simulink model "Aenea_model"  (R2020b)
settings: Solver=FixedStepDiscrete  StartTime=0.0  StopTime=10.0  FixedStep=0.02  RelTol=1e-3
undefined symbols (not defined in the file): attuatore_Amax, attuatore_Amin, attuatore_Emax, attuatore_Emin, attuatore_Rmax, attuatore_Rmin, attuatore_Tmax, attuatore_Tmin, bias, DiscIntNeverNeededParam, interventoA_05, interventoA_1, interventoE_05, interventoE_1, interventoT, inv_A, inv_comp_h, inv_E, inv_R, inv_T, K_AW_B_AP_quota, K_AW_B_becc, K_AW_B_imb, K_AW_B_roll, K_imb_inv, Kd_h_app, Kd_h_flare, Ki_AP_quota_select, Ki_AP_rotta, Ki_AP_vel, Ki_becch, Ki_h_app, Ki_h_cruise, Ki_h_flare, Ki_roll, Kp_AP_quota_hold_h, Kp_AP_quota_hold_l, Kp_AP_quota_select, Kp_AP_rotta, Kp_AP_vel, Kp_becch, Kp_comp_h, Kp_h_app_max, Kp_h_app_min, Kp_h_cruise, Kp_h_flare, Kp_imb, Kp_p, Kp_q, Kp_roll, Kp_Rotta_ATO, Newton, phi_max, phi_min, pwm_aileron_max, pwm_aileron_min, pwm_elevator_max, pwm_elevator_min, pwm_rudder_max, pwm_rudder_min ... (+19)
libraries: simulink_extras x41, slpidlib x8, simulink x6, dspsigops x4, arduinolib x3, svdutilitieslib x3, aerolibtransform2sys x2, aerolibtransform2 x2, aerosimlib x2, cstblocks x1
(part 5 of 7)

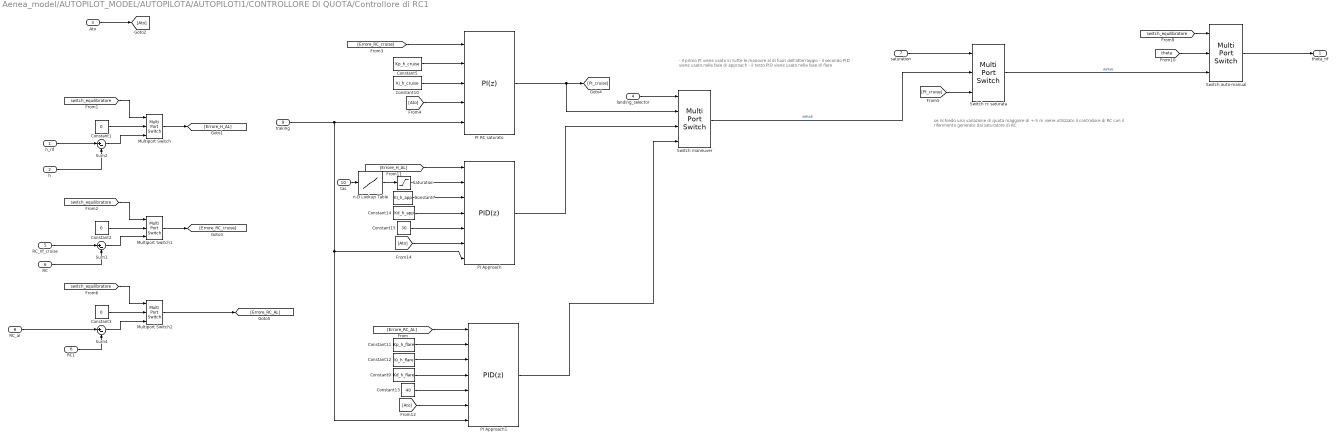
== system Aenea_model/AUTOPILOT_MODEL/AUTOPILOTA/AUTOPILOTI1/CONTROLLORE DI QUOTA/Controllore di RC1 ==
  note: - il primo PI viene usato in tutte le manovre al di fuori dell'atterraggio
      | - il secondo PID viene usato nella fase di approach
      | - il terzo PID viene usato nella fase di flare
  note: se richiedo una variazione di quota maggiore di +-5 m viene utilizzato il controllore di RC
      | con il riferimento generato dal saturatore di RC
  h_rif : Inport
  h : Inport  Port=2
  "Ato " : Inport  Port=3
  landing_selector : Inport  Port=4
  RC_rif_cruise : Inport  Port=5
  RC : Inport  Port=6
  saturation : Inport  Port=7
  "RC_al " : Inport  Port=8
  traking : Inport  Port=9
  tas : Inport  Port=10
  Constant1 : Constant  Value=0  SampleTime=t_AP
  Constant10 : Constant  Value=Ki_h_cruise  SampleTime=t_AP
  Constant11 : Constant  Value=Kp_h_flare  SampleTime=0.02
  Constant12 : Constant  Value=Ki_h_flare  SampleTime=0.02
  Constant13 : Constant  Value=40  SampleTime=0.02
  Constant14 : Constant  Value=Kd_h_app  SampleTime=0.02
  Constant15 : Constant  Value=30  SampleTime=0.02
  Constant2 : Constant  Value=0  SampleTime=t_AP
  Constant3 : Constant  Value=0  SampleTime=t_AP
  Constant5 : Constant  Value=Kp_h_cruise  SampleTime=t_AP
  Constant7 : Constant  Value=Ki_h_app  SampleTime=0.02
  Constant9 : Constant  Value=Kd_h_flare  SampleTime=0.02
  Multiport Switch : MultiPortSwitch  DataPortOrder=Zero-based contiguous  Inputs=2  zeroidx=on
  Multiport Switch1 : MultiPortSwitch  DataPortOrder=Zero-based contiguous  Inputs=2  zeroidx=on
  Multiport Switch2 : MultiPortSwitch  DataPortOrder=Zero-based contiguous  Inputs=2  zeroidx=on
  PI Approach : slpidlib/PID Controller  Controller=PID  Form=Parallel  TimeDomain=Discrete-time  UseExternalTs=off  SampleTime=0.02  IntegratorMethod=Forward Euler  FilterMethod=Forward Euler  ControllerParametersSource=external  P=1  I=1  D=0  UseFilter=on  N=100  TunerSelectOption=Transfer Function Based (PID Tuner App)  InitialConditionSource=internal  InitialConditionForIntegrator=0  InitialConditionForFilter=0  DifferentiatorICPrevScaledInput=0  ExternalReset=rising  TrackingMode=on  Kt=1  LimitOutput=off  SatLimitsSource=internal  UpperSaturationLimit=0.7  LowerSaturationLimit=-0.7  LinearizeAsGain=off  AntiWindupMode=back-calculation  Kb=1  POutMin=[]  POutMax=[]  IOutMin=[]  IOutMax=[]  DOutMin=[]  DOutMax=[]  NOutMin=[]  NOutMax=[]  SumOutMin=[]  SumOutMax=[]  SaturationOutMin=[]  SaturationOutMax=[]  PParamMin=[]  PParamMax=[]  IParamMin=[]  IParamMax=[]  DParamMin=[]  DParamMax=[]  NParamMin=[]  NParamMax=[]  KbParamMin=[]  KbParamMax=[]  KtParamMin=[]  KtParamMax=[]  KbOutMin=[]  KbOutMax=[]  KtOutMin=[]  KtOutMax=[]  IntegratorOutMin=[]  IntegratorOutMax=[]  FilterOutMin=[]  FilterOutMax=[]  SumI1OutMin=[]  SumI1OutMax=[]  SumI2OutMin=[]  SumI2OutMax=[]  SumI3OutMin=[]  SumI3OutMax=[]  SumI4OutMin=[]  SumI4OutMax=[]  SumDOutMin=[]  SumDOutMax=[]  DifferentiatorOutMin=[]  DifferentiatorOutMax=[]  FilterDiffOutCoefMin=[]  FilterDiffOutCoefMax=[]  ReciprocalOutMin=[]  ReciprocalOutMax=[]  SumDenOutMin=[]  SumDenOutMax=[]  SumNumOutMin=[]  SumNumOutMax=[]  DivideOutMin=[]  DivideOutMax=[]  UdiffTsProdOutMin=[]  UdiffTsProdOutMax=[]  NTsProdOutMin=[]  NTsProdOutMax=[]  UintegralTsProdOutMin=[]  UintegralTsProdOutMax=[]  UngainTsProdOutMin=[]  UngainTsProdOutMax=[]  IntegratorContinuousStateAttributes=''  IntegratorStateMustResolveToSignalObject=off  IntegratorRTWStateStorageClass=Auto  FilterContinuousStateAttributes=''  FilterStateMustResolveToSignalObject=off  FilterRTWStateStorageClass=Auto  ParallelPVariant=ExternalParameters  IdealPVariant=Disabled  IVariant=ExternalParameters  DVariant=ExternalParameters  IntegratorVariant=Discrete  SatVariant=Disabled  AWVariant=Passthrough  PCopyVariant=Disabled  TRVariant=Enabled  FdbkBlocksVariant=Forward  IdealPFdbkVariant=Disabled  SatFdbkVariant=Disabled  DerivativeFilterVariant=ForwardEulerFilter  NVariant=ExternalParameters  NCopyVariant=Disabled  FilterICVariant=InternalICsFilter  IntegratorICVariant=InternalICs  ExternalResetVariant=ExternalReset  TRSumVariant=TrackingMode  SumFdbkVariant=Disabled  SumVariant=Sum_PID  TsampFilterVariant=InternalTs  TsampNgainVariant=Passthrough  TsampIntegralVariant=Passthrough  ExternalSaturationOutDataTypeStr=Inherit: Same as second input
  PI Approach1 : slpidlib/PID Controller  Controller=PID  Form=Parallel  TimeDomain=Discrete-time  UseExternalTs=off  SampleTime=0.02  IntegratorMethod=Forward Euler  FilterMethod=Forward Euler  ControllerParametersSource=external  P=1  I=1  D=0  UseFilter=on  N=100  TunerSelectOption=Transfer Function Based (PID Tuner App)  InitialConditionSource=internal  InitialConditionForIntegrator=0  InitialConditionForFilter=0  DifferentiatorICPrevScaledInput=0  ExternalReset=rising  TrackingMode=on  Kt=1  LimitOutput=off  SatLimitsSource=internal  UpperSaturationLimit=0.7  LowerSaturationLimit=-0.7  LinearizeAsGain=off  AntiWindupMode=back-calculation  Kb=1  POutMin=[]  POutMax=[]  IOutMin=[]  IOutMax=[]  DOutMin=[]  DOutMax=[]  NOutMin=[]  NOutMax=[]  SumOutMin=[]  SumOutMax=[]  SaturationOutMin=[]  SaturationOutMax=[]  PParamMin=[]  PParamMax=[]  IParamMin=[]  IParamMax=[]  DParamMin=[]  DParamMax=[]  NParamMin=[]  NParamMax=[]  KbParamMin=[]  KbParamMax=[]  KtParamMin=[]  KtParamMax=[]  KbOutMin=[]  KbOutMax=[]  KtOutMin=[]  KtOutMax=[]  IntegratorOutMin=[]  IntegratorOutMax=[]  FilterOutMin=[]  FilterOutMax=[]  SumI1OutMin=[]  SumI1OutMax=[]  SumI2OutMin=[]  SumI2OutMax=[]  SumI3OutMin=[]  SumI3OutMax=[]  SumI4OutMin=[]  SumI4OutMax=[]  SumDOutMin=[]  SumDOutMax=[]  DifferentiatorOutMin=[]  DifferentiatorOutMax=[]  FilterDiffOutCoefMin=[]  FilterDiffOutCoefMax=[]  ReciprocalOutMin=[]  ReciprocalOutMax=[]  SumDenOutMin=[]  SumDenOutMax=[]  SumNumOutMin=[]  SumNumOutMax=[]  DivideOutMin=[]  DivideOutMax=[]  UdiffTsProdOutMin=[]  UdiffTsProdOutMax=[]  NTsProdOutMin=[]  NTsProdOutMax=[]  UintegralTsProdOutMin=[]  UintegralTsProdOutMax=[]  UngainTsProdOutMin=[]  UngainTsProdOutMax=[]  IntegratorContinuousStateAttributes=''  IntegratorStateMustResolveToSignalObject=off  IntegratorRTWStateStorageClass=Auto  FilterContinuousStateAttributes=''  FilterStateMustResolveToSignalObject=off  FilterRTWStateStorageClass=Auto  ParallelPVariant=ExternalParameters  IdealPVariant=Disabled  IVariant=ExternalParameters  DVariant=ExternalParameters  IntegratorVariant=Discrete  SatVariant=Disabled  AWVariant=Passthrough  PCopyVariant=Disabled  TRVariant=Enabled  FdbkBlocksVariant=Forward  IdealPFdbkVariant=Disabled  SatFdbkVariant=Disabled  DerivativeFilterVariant=ForwardEulerFilter  NVariant=ExternalParameters  NCopyVariant=Disabled  FilterICVariant=InternalICsFilter  IntegratorICVariant=InternalICs  ExternalResetVariant=ExternalReset  TRSumVariant=TrackingMode  SumFdbkVariant=Disabled  SumVariant=Sum_PID  TsampFilterVariant=InternalTs  TsampNgainVariant=Passthrough  TsampIntegralVariant=Passthrough  ExternalSaturationOutDataTypeStr=Inherit: Same as second input
  PI RC saturato : slpidlib/PID Controller  Controller=PI  Form=Parallel  TimeDomain=Discrete-time  UseExternalTs=off  SampleTime=0.02  IntegratorMethod=Forward Euler  FilterMethod=Forward Euler  ControllerParametersSource=external  P=1  I=1  D=0  UseFilter=on  N=100  TunerSelectOption=Transfer Function Based (PID Tuner App)  InitialConditionSource=internal  InitialConditionForIntegrator=0  InitialConditionForFilter=0  DifferentiatorICPrevScaledInput=0  ExternalReset=rising  TrackingMode=on  Kt=1  LimitOutput=off  SatLimitsSource=internal  UpperSaturationLimit=0.7  LowerSaturationLimit=-0.7  LinearizeAsGain=off  AntiWindupMode=back-calculation  Kb=1  POutMin=[]  POutMax=[]  IOutMin=[]  IOutMax=[]  DOutMin=[]  DOutMax=[]  NOutMin=[]  NOutMax=[]  SumOutMin=[]  SumOutMax=[]  SaturationOutMin=[]  SaturationOutMax=[]  PParamMin=[]  PParamMax=[]  IParamMin=[]  IParamMax=[]  DParamMin=[]  DParamMax=[]  NParamMin=[]  NParamMax=[]  KbParamMin=[]  KbParamMax=[]  KtParamMin=[]  KtParamMax=[]  KbOutMin=[]  KbOutMax=[]  KtOutMin=[]  KtOutMax=[]  IntegratorOutMin=[]  IntegratorOutMax=[]  FilterOutMin=[]  FilterOutMax=[]  SumI1OutMin=[]  SumI1OutMax=[]  SumI2OutMin=[]  SumI2OutMax=[]  SumI3OutMin=[]  SumI3OutMax=[]  SumI4OutMin=[]  SumI4OutMax=[]  SumDOutMin=[]  SumDOutMax=[]  DifferentiatorOutMin=[]  DifferentiatorOutMax=[]  FilterDiffOutCoefMin=[]  FilterDiffOutCoefMax=[]  ReciprocalOutMin=[]  ReciprocalOutMax=[]  SumDenOutMin=[]  SumDenOutMax=[]  SumNumOutMin=[]  SumNumOutMax=[]  DivideOutMin=[]  DivideOutMax=[]  UdiffTsProdOutMin=[]  UdiffTsProdOutMax=[]  NTsProdOutMin=[]  NTsProdOutMax=[]  UintegralTsProdOutMin=[]  UintegralTsProdOutMax=[]  UngainTsProdOutMin=[]  UngainTsProdOutMax=[]  IntegratorContinuousStateAttributes=''  IntegratorStateMustResolveToSignalObject=off  IntegratorRTWStateStorageClass=Auto  FilterContinuousStateAttributes=''  FilterStateMustResolveToSignalObject=off  FilterRTWStateStorageClass=Auto  ParallelPVariant=ExternalParameters  IdealPVariant=Disabled  IVariant=ExternalParameters  DVariant=Disabled  IntegratorVariant=Discrete  SatVariant=Disabled  AWVariant=Passthrough  PCopyVariant=Disabled  TRVariant=Enabled  FdbkBlocksVariant=Forward  IdealPFdbkVariant=Disabled  SatFdbkVariant=Disabled  DerivativeFilterVariant=Disabled  NVariant=Disabled  NCopyVariant=Disabled_SignalSpec  FilterICVariant=Disabled  IntegratorICVariant=InternalICs  ExternalResetVariant=ExternalReset  TRSumVariant=TrackingMode  SumFdbkVariant=Disabled  SumVariant=Sum_PI  TsampFilterVariant=InternalTs  TsampNgainVariant=Passthrough  TsampIntegralVariant=Passthrough  ExternalSaturationOutDataTypeStr=Inherit: Same as second input
  RC1 : InportShadow  Port=6
  Saturation : Saturate  UpperLimit=0.046  LowerLimit=0.01
  Sum1 : Sum  Inputs=|+-
  Sum2 : Sum  Inputs=|+-
  Sum4 : Sum  Inputs=|+-
  Switch auto-manual : MultiPortSwitch  DataPortOrder=Zero-based contiguous  Inputs=2  zeroidx=on
  Switch maneuver : MultiPortSwitch  DataPortOrder=Zero-based contiguous  zeroidx=on
  Switch rc saturata : MultiPortSwitch  DataPortOrder=Zero-based contiguous  Inputs=2  zeroidx=on
  n-D Lookup Table : Lookup_n-D  NumberOfTableDimensions=1  BreakpointsForDimension1="[V_stall*1.2  V_max*0.75]"  Table=[Kp_h_app_max Kp_h_app_min]  RndMeth=Simplest  InputSameDT=on
  theta_rif : Outport  VectorParamsAs1DForOutWhenUnconnected=off
  wires:
  landing_selector/1 -> Switch maneuver/1
  [Ato] -> PI Approach/6
  "Ato "/1 -> [Ato]
  [Errore_H_AL] -> PI Approach/1
  [switch_equilibratore] -> Switch auto-manual/1
  [theta] -> Switch auto-manual/2
  Multiport Switch/1 -> [Errore_H_AL]
  [switch_equilibratore] -> Multiport Switch/1
  Constant1/1 -> Multiport Switch/2
  Sum2/1 -> Multiport Switch/3
  h/1 -> Sum2/2
  h_rif/1 -> Sum2/1
  Saturation/1 -> PI Approach/2
  Constant7/1 -> PI Approach/3
  RC_rif_cruise/1 -> Sum1/1
  Sum1/1 -> Multiport Switch1/3
  Constant2/1 -> Multiport Switch1/2
  Multiport Switch1/1 -> [Errore_RC_cruise]
  [switch_equilibratore] -> Multiport Switch1/1
  Switch maneuver/1 -> Switch rc saturata/2  "deltaE"
  RC/1 -> Sum1/2
  saturation/1 -> Switch rc saturata/1
  Switch rc saturata/1 -> Switch auto-manual/3  "deltaE"
  PI RC saturato/1 -> [PI_cruise], Switch maneuver/2
  Constant5/1 -> PI RC saturato/2
  [Ato] -> PI RC saturato/4
  Constant10/1 -> PI RC saturato/3
  [Errore_RC_cruise] -> PI RC saturato/1
  [PI_cruise] -> Switch rc saturata/3
  "RC_al "/1 -> Sum4/1
  [switch_equilibratore] -> Multiport Switch2/1
  RC1/1 -> Sum4/2
  Multiport Switch2/1 -> [Errore_RC_AL]
  Constant3/1 -> Multiport Switch2/2
  Sum4/1 -> Multiport Switch2/3
  PI Approach/1 -> Switch maneuver/3
  [Errore_RC_AL] -> PI Approach1/1
  Constant11/1 -> PI Approach1/2
  Constant12/1 -> PI Approach1/3
  [Ato] -> PI Approach1/6
  Switch auto-manual/1 -> theta_rif/1
  PI Approach1/1 -> Switch maneuver/4
  traking/1 -> PI Approach1/7, PI Approach/7, PI RC saturato/5
  Constant9/1 -> PI Approach1/4
  Constant13/1 -> PI Approach1/5
  Constant14/1 -> PI Approach/4
  Constant15/1 -> PI Approach/5
  tas/1 -> n-D Lookup Table/1
  n-D Lookup Table/1 -> Saturation/1

== system Aenea_model/AUTOPILOT_MODEL/AUTOPILOTA/AUTOPILOTI1/CONTROLLORE DI QUOTA/Saturazione RC  ==
  V : Inport
  RC : Inport  Port=2
  Constant : Constant  Value=-5  SampleTime=t_AP
  Lookup Table2 : Lookup  InputValues=[15;20;25;30;35;40]  Table=[2;2.5;3;3.5;4;4]
  Saturation Dynamic1 : simulink/Discontinuities/Saturation Dynamic  OutMin=[]  OutMax=[]  OutDataTypeStr=Inherit: Same as second input  OutDataType=fixdt(1, 16)  OutScaling=2^-10  DoSatur=off
  RC_verficata : Outport  VectorParamsAs1DForOutWhenUnconnected=off
  wires:
  V/1 -> Lookup Table2/1
  RC/1 -> Saturation Dynamic1/2
  Lookup Table2/1 -> Saturation Dynamic1/1
  Constant/1 -> Saturation Dynamic1/3
  Saturation Dynamic1/1 -> RC_verficata/1

== system Aenea_model/AUTOPILOT_MODEL/AUTOPILOTA/AUTOPILOTI1/CONTROLLORE DI ROTTA/ATO ==
  In1 : Inport
  In2 : Inport  Port=2
  In3 : Inport  Port=3
  In4 : Inport  Port=4
  Constant3 : Constant  Value=Kp_Rotta_ATO
  Constant4 : Constant  Value=0
  Multiport Switch2 : MultiPortSwitch  DataPortOrder=Zero-based contiguous  Inputs=2  zeroidx=on
  Multiport Switch3 : MultiPortSwitch  DataPortOrder=Zero-based contiguous  Inputs=2  zeroidx=on
  Switch3 : Switch  Criteria=u2 > Threshold  Threshold=2
  Switch4 : Switch  Criteria=u2 > Threshold  Threshold=2
  Out1 : Outport  VectorParamsAs1DForOutWhenUnconnected=off
  Out2 : Outport  Port=2  VectorParamsAs1DForOutWhenUnconnected=off
  wires:
  Switch3/1 -> Out1/1
  Constant4/1 -> Multiport Switch3/3
  In1/1 -> Switch3/1, Multiport Switch2/2
  [Switch_ATO] -> Multiport Switch3/1
  [Alt] -> Switch3/2
  Multiport Switch2/1 -> Switch3/3
  [Alt] -> Switch4/2
  [Switch_ATO] -> Multiport Switch2/1
  In4/1 -> Switch4/1, Multiport Switch3/2
  Constant3/1 -> Multiport Switch2/3
  Switch4/1 -> Out2/1
  In2/1 -> [Switch_ATO]
  In3/1 -> [Alt]
  Multiport Switch3/1 -> Switch4/3

== system Aenea_model/AUTOPILOT_MODEL/AUTOPILOTA/AUTOPILOTI1/CONTROLLORE DI ROTTA/calcolo errore Psi  ==
  psi_ref (°) : Inport
  psi (rad) : Inport  Port=2
  Constant : Constant  Value=360  SampleTime=t_AP
  Constant1 : Constant  Value=360  SampleTime=t_AP
  Constant2 : Constant  Value=360  SampleTime=t_AP
  Degrees to Radians : simulink_extras/Transformations/Degrees to Radians
  Math Function : Math  Operator=mod  SignedPower=on  SaturateOnIntegerOverflow=on
  Radians to Degrees : simulink_extras/Transformations/Radians to Degrees
  Sum : Sum  Inputs=|+-
  Sum1 : Sum  Inputs=|+-
  Sum2 : Sum  Inputs=|++
  Switch : Switch  Threshold=180
  Switch1 : Switch  Threshold=-180
  psi_err : Outport  VectorParamsAs1DForOutWhenUnconnected=off
  wires:
  Radians to Degrees/1 -> Math Function/1
  Degrees to Radians/1 -> psi_err/1
  Switch1/1 -> Degrees to Radians/1
  Sum2/1 -> Switch1/3
  Constant2/1 -> Sum2/2
  Switch/1 -> Switch1/1
  Sum/1 -> Sum2/1, Switch1/2, Switch/3, Switch/2, Sum1/1
  Constant1/1 -> Sum1/2
  Sum1/1 -> Switch/1
  Math Function/1 -> Sum/2
  Constant/1 -> Math Function/2
  psi (rad)/1 -> Radians to Degrees/1
  psi_ref (°)/1 -> Sum/1

== system Aenea_model/AUTOPILOT_MODEL/AUTOPILOTA/AUTOPILOTI1/CONTROLLORE DI VELOCITA'/Smooth Switch ==
  switch_manetta : Inport
  manetta_manuale : Inport  Port=2
  manetta_controllo : Inport  Port=3
  Buffer : Buffer  N=2  OutputFrames=off
  Delay : Delay  DelayLength=1
  Digital Clock1 : DigitalClock  SampleTime=0.02
  Smooth Bypass : MATLAB Function  TreatAsAtomicUnit=on
  Switch Bumpless 1 : MultiPortSwitch  DataPortOrder=Zero-based contiguous  Inputs=2  zeroidx=on
  Vector Concatenate : Concatenate
  Out1 : Outport
  wires:
  Delay/1 -> Vector Concatenate/2
  switch_manetta/1 -> Switch Bumpless 1/1, Smooth Bypass/2(switch_manetta), Vector Concatenate/1
  Smooth Bypass/1(y) -> Switch Bumpless 1/3
  manetta_manuale/1 -> Switch Bumpless 1/2, Smooth Bypass/4(u)
  Buffer/1 -> Smooth Bypass/1(buffer)
  Digital Clock1/1 -> Smooth Bypass/3(clock)
  Smooth Bypass/2(clock_init) -> Delay/1
  Vector Concatenate/1 -> Buffer/1
  manetta_controllo/1 -> Smooth Bypass/5(u_filt)
  Switch Bumpless 1/1 -> Out1/1

== system Aenea_model/AUTOPILOT_MODEL/AUTOPILOTA/AUTOPILOTI1/CONTROLLORE DI VELOCITA'/throttle - landing ==
  AL : Inport
  In2 : Inport  Port=2
  Alt : Inport  Port=3
  Constant3 : Constant  Value=0
  Enabled Subsystem : Subsystem  TreatAsAtomicUnit=on
  Hit Crossing : HitCross  HitCrossingOffset=0.3  HitCrossingDirection=falling
  Switch : Switch  Criteria=u2 > Threshold
  throttle - landing : MultiPortSwitch  DataPortOrder=Zero-based contiguous  Inputs=2  zeroidx=on
  Out1 : Outport  VectorParamsAs1DForOutWhenUnconnected=off
  wires:
  Switch/1 -> throttle - landing/3
  throttle - landing/1 -> Out1/1
  AL/1 -> throttle - landing/1
  Alt/1 -> Hit Crossing/1
  In2/1 -> Switch/1, throttle - landing/2
  Constant3/1 -> Switch/3
  Hit Crossing/1 -> Enabled Subsystem/Trigger
  Enabled Subsystem/1(Out1) -> Switch/2

== system Aenea_model/AUTOPILOT_MODEL/AUTOPILOTA/CONTROLLI INTERNI E SWITCH1/Controllore PID/elevator - landing ==
  In1 : Inport
  Tas : Inport  Port=2
  AL : Inport  Port=3
  Constant5 : Constant  Value=0
  Multiport Switch2 : MultiPortSwitch  DataPortOrder=Zero-based contiguous  Inputs=2  zeroidx=on
  Switch1 : Switch  Threshold=16
  Out1 : Outport  VectorParamsAs1DForOutWhenUnconnected=off
  wires:
  Multiport Switch2/1 -> Out1/1
  Tas/1 -> Switch1/2
  In1/1 -> Multiport Switch2/2, Switch1/1
  AL/1 -> Multiport Switch2/1
  Constant5/1 -> Switch1/3
  Switch1/1 -> Multiport Switch2/3

== system Aenea_model/AUTOPILOT_MODEL/AUTOPILOTA/CONTROLLI INTERNI E SWITCH1/Controllore PID/elevator - takeoff ==
  In1 : Inport
  Fase_ATO : Inport  Port=2
  ATO : Inport  Port=3
  eq_rot : Inport  Port=4
  Degrees to Radians : simulink_extras/Transformations/Degrees to Radians
  Multiport Switch1 : MultiPortSwitch  DataPortOrder=Zero-based contiguous  Inputs=5  zeroidx=on
  Multiport Switch2 : MultiPortSwitch  DataPortOrder=Zero-based contiguous  Inputs=2  zeroidx=on
  Out1 : Outport  VectorParamsAs1DForOutWhenUnconnected=off
  wires:
  ATO/1 -> Multiport Switch2/1
  In1/1 -> Multiport Switch1/6, Multiport Switch1/5, Multiport Switch2/2
  Multiport Switch2/1 -> Out1/1
  Multiport Switch1/1 -> Multiport Switch2/3
  Fase_ATO/1 -> Multiport Switch1/1
  eq_rot/1 -> Degrees to Radians/1
  Degrees to Radians/1 -> Multiport Switch1/4, Multiport Switch1/3, Multiport Switch1/2

== system Aenea_model/AUTOPILOT_MODEL/AUTOPILOTA/GESTIONE AUTOPILOTI1/Interruttore_Intervento/Enabled Subsystem ==
  Time : Inport
  Enable : EnablePort
  Constant1 : Constant  Value=0
  Constant2 : Constant
  Switch : Switch  Criteria=u2 > Threshold  Threshold=2
  1/0 : Outport  VectorParamsAs1DForOutWhenUnconnected=off
  wires:
  Time/1 -> Switch/2
  Constant1/1 -> Switch/1
  Constant2/1 -> Switch/3
  Switch/1 -> 1/0/1

== system Aenea_model/AUTOPILOT_MODEL/AUTOPILOTA/GESTIONE AUTOPILOTI1/Interruttore_Intervento/Resettable Subsystem ==
  Reset : ResetPort  DisableCoverage=on
  CLOCK : Subsystem
  Time : Outport  VectorParamsAs1DForOutWhenUnconnected=off
  wires:
  CLOCK/1(Time) -> Time/1

== system Aenea_model/AUTOPILOT_MODEL/AUTOPILOTA/GESTIONE AUTOPILOTI1/Interruttore_Safe/Enabled Subsystem ==
  Time : Inport
  Enable : EnablePort
  Constant1 : Constant  Value=0
  Constant2 : Constant
  Switch : Switch  Criteria=u2 > Threshold  Threshold=2
  1/0 : Outport  VectorParamsAs1DForOutWhenUnconnected=off
  wires:
  Time/1 -> Switch/2
  Constant1/1 -> Switch/1
  Constant2/1 -> Switch/3
  Switch/1 -> 1/0/1

== system Aenea_model/AUTOPILOT_MODEL/AUTOPILOTA/GESTIONE AUTOPILOTI1/Interruttore_Safe/Resettable Subsystem ==
  Reset : ResetPort  DisableCoverage=on
  CLOCK : Subsystem
  Time : Outport  VectorParamsAs1DForOutWhenUnconnected=off
  wires:
  CLOCK/1(Time) -> Time/1

== system Aenea_model/AUTOPILOT_MODEL/AUTOPILOTA/GESTIONE AUTOPILOTI1/Intervento Manager/Alarm_Timing_0.5sec ==
  Intervento_IN : Inport
  "Enabled " : Subsystem  TreatAsAtomicUnit=on
  Resettable Subsystem : Subsystem  TreatAsAtomicUnit=on
  Alarm : Outport  VectorParamsAs1DForOutWhenUnconnected=off
  wires:
  Intervento_IN/1 -> Resettable Subsystem/Reset, "Enabled "/Enable
  Resettable Subsystem/1(Time) -> "Enabled "/1("Time ")
  "Enabled "/1(Alarm_Int) -> Alarm/1

== system Aenea_model/AUTOPILOT_MODEL/AUTOPILOTA/GESTIONE AUTOPILOTI1/Intervento Manager/Alarm_Timing_1sec ==
  Intervento_IN : Inport
  "Enabled " : Subsystem  TreatAsAtomicUnit=on
  Resettable Subsystem : Subsystem  TreatAsAtomicUnit=on
  Alarm : Outport  VectorParamsAs1DForOutWhenUnconnected=off
  wires:
  Intervento_IN/1 -> Resettable Subsystem/Reset, "Enabled "/Enable
  Resettable Subsystem/1(Time) -> "Enabled "/1("Time ")
  "Enabled "/1(Alarm_Int) -> Alarm/1

== system Aenea_model/AUTOPILOT_MODEL/AUTOPILOTA/GESTIONE AUTOPILOTI1/Safe Manager/Alarm_Timing ==
  Alarm_IN : Inport
  "Enabled " : Subsystem  TreatAsAtomicUnit=on
  Resettable Subsystem : Subsystem  TreatAsAtomicUnit=on
  Alarm : Outport  VectorParamsAs1DForOutWhenUnconnected=off
  wires:
  Alarm_IN/1 -> Resettable Subsystem/Reset, "Enabled "/Enable
  Resettable Subsystem/1(Time) -> "Enabled "/1("Time ")
  "Enabled "/1(Alarm Safe) -> Alarm/1

== system Aenea_model/AUTOPILOT_MODEL/AUTOPILOTA/Subsystem1/Subsystem1/APPROACH ==
  dist : Inport
  h_g : Inport  Port=2
  x_g : Inport  Port=3
  V_ : Inport  Port=4
  Enable : EnablePort  ShowOutputPort=on
  Abs : Abs
  Atan : Trigonometry  Operator=atan
  Constant1 : Constant  Value=20  SampleTime=0.02
  Constant2 : Constant  SampleTime=0.02
  Constant3 : Constant  SampleTime=0.02
  Constant4 : Constant  Value=0  SampleTime=0.02
  Discrete-Time Integrator : DiscreteIntegrator  gainval=1  ExternalReset=rising  SampleTime=0.02  LimitOutput=on  UpperSaturationLimit=1  LowerSaturationLimit=0  ICPrevOutput=DiscIntNeverNeededParam  ICPrevScaledInput=DiscIntNeverNeededParam
  Divide : Product  Inputs=*/
  Gain : Gain  Gain=-1
  MATLAB Function : MATLAB Function  TreatAsAtomicUnit=on
  Multiply : Product
  Multiply1 : Product
  Mux : Mux
  Sum : Sum  Inputs=|+-
  Sum1 : Sum  Inputs=|+-
  Switch : Switch  Criteria=u2 > Threshold
  x_g0 : Constant  Value=-100  SampleTime=0.02
  h_ref : Outport  VectorParamsAs1DForOutWhenUnconnected=off
  V1 : Outport  Port=2  VectorParamsAs1DForOutWhenUnconnected=off
  flare_data : Outport  Port=3  VectorParamsAs1DForOutWhenUnconnected=off
  landing_abort : Outport  Port=4  VectorParamsAs1DForOutWhenUnconnected=off
  rc_ref_app : Outport  Port=5  VectorParamsAs1DForOutWhenUnconnected=off
  wires:
  Constant1/1 -> V1/1
  h_g/1 -> Divide/1
  Sum/1 -> Divide/2
  x_g/1 -> Sum/1
  Sum1/1 -> Gain/1
  Gain/1 -> Multiply/2
  dist/1 -> Sum1/1
  x_g0/1 -> Sum/2, MATLAB Function/3(xg0), Sum1/2
  Multiply/1 -> h_ref/1
  Mux/1 -> flare_data/1
  MATLAB Function/2(h_f_out) -> Mux/2
  MATLAB Function/1(x_f_out) -> Mux/1
  Abs/1 -> MATLAB Function/2(gamma)
  MATLAB Function/3(k_x_out) -> Mux/3
  MATLAB Function/4(h_c_out) -> Mux/4
  MATLAB Function/5(no_solution) -> landing_abort/1
  Constant2/1 -> Discrete-Time Integrator/1
  Constant3/1 -> Switch/1
  Enable/1 -> Discrete-Time Integrator/2
  Constant4/1 -> Switch/3
  Discrete-Time Integrator/1 -> Switch/2
  Switch/1 -> MATLAB Function/1(reset)
  V_/1 -> Multiply1/1
  Multiply1/1 -> rc_ref_app/1
  Divide/1 -> Multiply1/2, Multiply/1, Atan/1
  Atan/1 -> Abs/1

== system Aenea_model/AUTOPILOT_MODEL/AUTOPILOTA/Subsystem1/Subsystem1/CREAZIONE_WAYPOINT  ==
  Lat_Home : Inport
  Long_Home : Inport  Port=2
  h_Home : Inport  Port=3
  psi_Home : Inport  Port=4
  AUTOLANDING_WAYPOINTS : MATLAB Function  TreatAsAtomicUnit=on
  Constant : Constant  Value=vel_wp1_al
  Constant1 : Constant  Value=vel_wp2_al
  MATLAB Function : MATLAB Function  TreatAsAtomicUnit=on
  Radians to Degrees : simulink_extras/Transformations/Radians to Degrees
  Radians to Degrees1 : simulink_extras/Transformations/Radians to Degrees
  alt waypoint virtuale : Constant  Value=[45 45 45]
  distance waypoints virtuale : Constant  Value=[-1000 -800 2000]
  WP_info : Outport  VectorParamsAs1DForOutWhenUnconnected=off
  WP_param : Outport  Port=2  VectorParamsAs1DForOutWhenUnconnected=off
  wires:
  alt waypoint virtuale/1 -> AUTOLANDING_WAYPOINTS/4(alt)
  distance waypoints virtuale/1 -> MATLAB Function/4(distance)
  Lat_Home/1 -> MATLAB Function/1(lat_ini)
  Long_Home/1 -> MATLAB Function/2(long_ini)
  psi_Home/1 -> MATLAB Function/3(heading)
  h_Home/1 -> AUTOLANDING_WAYPOINTS/3(h_Home)
  MATLAB Function/1(lat_end) -> Radians to Degrees/1
  MATLAB Function/2(long_end) -> Radians to Degrees1/1
  Radians to Degrees/1 -> AUTOLANDING_WAYPOINTS/1(Lat_Home)
  Radians to Degrees1/1 -> AUTOLANDING_WAYPOINTS/2(Long_Home)
  AUTOLANDING_WAYPOINTS/1(WP_info) -> WP_info/1
  AUTOLANDING_WAYPOINTS/2(WP_param) -> WP_param/1
  Constant/1 -> AUTOLANDING_WAYPOINTS/5(vel_wp1_al)
  Constant1/1 -> AUTOLANDING_WAYPOINTS/6(vel_wp2_al)

== system Aenea_model/AUTOPILOT_MODEL/AUTOPILOTA/Subsystem1/Subsystem1/FLARE ==
  x_e : Inport
  flare_data : Inport  Port=2
  V_ : Inport  Port=3
  Enable : EnablePort
  Constant1 : Constant  Value=18  SampleTime=0.02
  Demux : Demux
  Exp : Math  SignedPower=on  SaturateOnIntegerOverflow=on
  Exp1 : Math  SignedPower=on  SaturateOnIntegerOverflow=on
  Gain : Gain  Gain=-1
  Gain1 : Gain  Gain=-1
  Gain2 : Gain  Gain=-1
  MATLAB Function : MATLAB Function  Commented=on  TreatAsAtomicUnit=on
  Multiply{,1..3} (4 alike) : Product
  Multiply4 : Product  Inputs=3
  Sum{,1,3..4} (4 alike) : Sum  Inputs=|+-
  Sum2 : Sum  Inputs=|++
  x_e1 : InportShadow
  Tas_ref1 : Outport  VectorParamsAs1DForOutWhenUnconnected=off
  h_ref : Outport  Port=2  VectorParamsAs1DForOutWhenUnconnected=off
  RC_ref : Outport  Port=3  VectorParamsAs1DForOutWhenUnconnected=off
  wires:
  MATLAB Function/1(rotta) -> ?
  Constant1/1 -> Tas_ref1/1
  x_e/1 -> Sum/1
  Sum/1 -> Multiply/1
  Multiply/1 -> Gain/1
  Gain/1 -> Exp/1
  Exp/1 -> Multiply1/1
  Sum1/1 -> Multiply1/2
  Multiply1/1 -> Sum2/1
  flare_data/1 -> Demux/1
  Sum2/1 -> h_ref/1
  Gain1/1 -> Exp1/1
  Demux/1 -> Sum3/2, Sum/2  "x_f"
  Demux/2 -> Sum4/1, Sum1/1  "h_f"
  x_e1/1 -> Sum3/1
  Exp1/1 -> Multiply3/1
  Gain2/1 -> RC_ref/1
  Demux/4 -> Sum4/2, Sum1/2, Sum2/2  "h_c"
  Multiply2/1 -> Gain1/1
  Sum3/1 -> Multiply2/1
  Demux/3 -> Multiply2/2, Multiply4/3, Multiply/2  "k_x"
  Multiply3/1 -> Gain2/1
  Sum4/1 -> Multiply4/1
  V_/1 -> Multiply4/2
  Multiply4/1 -> Multiply3/2

== system Aenea_model/AUTOPILOT_MODEL/AUTOPILOTA/Subsystem1/Subsystem1/INSEGUIMENTO CENTRO PISTA ==
  y_e : Inport
  psi_home : Inport  Port=2
  Enable : EnablePort
  Gain1 : Gain
  PID Controller : slpidlib/PID Controller  Controller=PI  Form=Parallel  TimeDomain=Discrete-time  UseExternalTs=off  SampleTime=-1  IntegratorMethod=Forward Euler  FilterMethod=Forward Euler  ControllerParametersSource=external  P=1  I=1  D=0  UseFilter=on  N=100  TunerSelectOption=Transfer Function Based (PID Tuner App)  InitialConditionSource=internal  InitialConditionForIntegrator=0  InitialConditionForFilter=0  DifferentiatorICPrevScaledInput=0  ExternalReset=none  TrackingMode=off  Kt=1  LimitOutput=off  SatLimitsSource=internal  UpperSaturationLimit=inf  LowerSaturationLimit=-inf  LinearizeAsGain=on  AntiWindupMode=none  Kb=1  POutMin=[]  POutMax=[]  IOutMin=[]  IOutMax=[]  DOutMin=[]  DOutMax=[]  NOutMin=[]  NOutMax=[]  SumOutMin=[]  SumOutMax=[]  SaturationOutMin=[]  SaturationOutMax=[]  PParamMin=[]  PParamMax=[]  IParamMin=[]  IParamMax=[]  DParamMin=[]  DParamMax=[]  NParamMin=[]  NParamMax=[]  KbParamMin=[]  KbParamMax=[]  KtParamMin=[]  KtParamMax=[]  KbOutMin=[]  KbOutMax=[]  KtOutMin=[]  KtOutMax=[]  IntegratorOutMin=[]  IntegratorOutMax=[]  FilterOutMin=[]  FilterOutMax=[]  SumI1OutMin=[]  SumI1OutMax=[]  SumI2OutMin=[]  SumI2OutMax=[]  SumI3OutMin=[]  SumI3OutMax=[]  SumI4OutMin=[]  SumI4OutMax=[]  SumDOutMin=[]  SumDOutMax=[]  DifferentiatorOutMin=[]  DifferentiatorOutMax=[]  FilterDiffOutCoefMin=[]  FilterDiffOutCoefMax=[]  ReciprocalOutMin=[]  ReciprocalOutMax=[]  SumDenOutMin=[]  SumDenOutMax=[]  SumNumOutMin=[]  SumNumOutMax=[]  DivideOutMin=[]  DivideOutMax=[]  UdiffTsProdOutMin=[]  UdiffTsProdOutMax=[]  NTsProdOutMin=[]  NTsProdOutMax=[]  UintegralTsProdOutMin=[]  UintegralTsProdOutMax=[]  UngainTsProdOutMin=[]  UngainTsProdOutMax=[]  IntegratorContinuousStateAttributes=''  IntegratorStateMustResolveToSignalObject=off  IntegratorRTWStateStorageClass=Auto  FilterContinuousStateAttributes=''  FilterStateMustResolveToSignalObject=off  FilterRTWStateStorageClass=Auto  ParallelPVariant=ExternalParameters  IdealPVariant=Disabled  IVariant=ExternalParameters  DVariant=Disabled  IntegratorVariant=Discrete  SatVariant=Disabled  AWVariant=Passthrough  PCopyVariant=Disabled  TRVariant=Disabled  FdbkBlocksVariant=Forward  IdealPFdbkVariant=Disabled  SatFdbkVariant=Disabled  DerivativeFilterVariant=Disabled  NVariant=Disabled  NCopyVariant=Disabled_SignalSpec  FilterICVariant=Disabled  IntegratorICVariant=InternalICs  ExternalResetVariant=Disabled  TRSumVariant=Passthrough  SumFdbkVariant=Disabled  SumVariant=Sum_PI  TsampFilterVariant=InternalTs  TsampNgainVariant=Passthrough  TsampIntegralVariant=Passthrough  ExternalSaturationOutDataTypeStr=Inherit: Same as second input
  Radians to Degrees2 : simulink_extras/Transformations/Radians to Degrees
  Sum3 : Sum  Inputs=|+-
  psi ref gain : Constant  Value=0.0052  SampleTime=t_AP
  psi ref gain1 : Constant  Value=0.00052  SampleTime=t_AP
  psi_ref_landing : Outport  VectorParamsAs1DForOutWhenUnconnected=off
  wires:
  psi_home/1 -> [psi_home]
  y_e/1 -> Gain1/1
  Gain1/1 -> PID Controller/1
  psi ref gain/1 -> PID Controller/2
  [psi_home] -> Sum3/1
  Sum3/1 -> Radians to Degrees2/1
  Radians to Degrees2/1 -> psi_ref_landing/1
  psi ref gain1/1 -> PID Controller/3
  PID Controller/1 -> Sum3/2

== system Aenea_model/AUTOPILOT_MODEL/AUTOPILOTA/Subsystem1/Subsystem1/LLA to Flat Earth ==
  latlong : Inport
  h : Inport  Port=2
  ground height : Inport  Port=3
  latlong_ref : Inport  Port=4
  psi_ref : Inport  Port=5
  Degrees to Radians : simulink_extras/Transformations/Degrees to Radians
  LatLong wrap : aerolibtransform2sys/LatLong wrap  SystemSampleTime=-1  VariantActivationTime=update diagram  Latency=0  AutoFrameSizeCalculation=off
      settings: SourceProductBaseCode=AE
  LatLong wrap LL0 : aerolibtransform2sys/LatLong wrap  SystemSampleTime=-1  VariantActivationTime=update diagram  Latency=0  AutoFrameSizeCalculation=off
      settings: SourceProductBaseCode=AE
  Mux : Mux  Inputs=3
  Subsystem1 : Subsystem
  Sum : Sum  Inputs=++|
  Sum1 : Sum  Inputs=|+-
  Ze2height : UnaryMinus
  initial_latg : Selector  InputPortWidth=2  IndexOptions=Index vector (dialog)  Indices=[1]  OutputSizes=1
  Xe : Outport  VectorParamsAs1DForOutWhenUnconnected=off
  wires:
  Degrees to Radians/1 -> Subsystem1/1(pos_rad)
  initial_latg/1 -> Subsystem1/2(mu)
  ground height/1 -> Sum/2
  LatLong wrap/1 -> Degrees to Radians/1
  LatLong wrap LL0/1 -> Sum1/2, initial_latg/1
  Sum1/1 -> LatLong wrap/1
  Ze2height/1 -> Mux/3  "Pz"
  Subsystem1/1(Px) -> Mux/1
  Subsystem1/2(Py) -> Mux/2
  Mux/1 -> Xe/1
  latlong_ref/1 -> LatLong wrap LL0/1
  Sum/1 -> Ze2height/1  "alt"
  h/1 -> Sum/1
  psi_ref/1 -> Subsystem1/3(psi_ref)
  latlong/1 -> Sum1/1

== system Aenea_model/AUTOPILOT_MODEL/Misure Sensori/BMP_280/Subsystem/Subsystem1 ==
  T : Inport
  Enable : EnablePort
  T_0 : Outport  VectorParamsAs1DForOutWhenUnconnected=off
  wires:
  T/1 -> T_0/1

== system Aenea_model/AUTOPILOT_MODEL/AUTOPILOTA/AUTOPILOTI1/CONTROLLORE DI VELOCITA'/throttle - landing/Enabled Subsystem ==
  Trigger : TriggerPort  VariantControl=Variant  PortDimensions=1
  Constant : Constant  Value=0
  Out1 : Outport  InitialOutput=[1]  VectorParamsAs1DForOutWhenUnconnected=off
  wires:
  Constant/1 -> Out1/1

== system Aenea_model/AUTOPILOT_MODEL/AUTOPILOTA/GESTIONE AUTOPILOTI1/Interruttore_Intervento/Resettable Subsystem/CLOCK ==
  Constant4 : Constant  Value=t_AP  SampleTime=t_AP
  Memory : Memory  InheritSampleTime=on
  Sum : Sum  Inputs=|++
  Time : Outport  VectorParamsAs1DForOutWhenUnconnected=off
  wires:
  Memory/1 -> Sum/2
  Sum/1 -> Memory/1, Time/1
  Constant4/1 -> Sum/1

== system Aenea_model/AUTOPILOT_MODEL/AUTOPILOTA/GESTIONE AUTOPILOTI1/Interruttore_Safe/Resettable Subsystem/CLOCK ==
  Constant4 : Constant  Value=t_AP  SampleTime=t_AP
  Memory : Memory  InheritSampleTime=on
  Sum : Sum  Inputs=|++
  Time : Outport  VectorParamsAs1DForOutWhenUnconnected=off
  wires:
  Memory/1 -> Sum/2
  Sum/1 -> Memory/1, Time/1
  Constant4/1 -> Sum/1

== system Aenea_model/AUTOPILOT_MODEL/AUTOPILOTA/GESTIONE AUTOPILOTI1/Intervento Manager/Alarm_Timing_0.5sec/Enabled  ==
  "Time " : Inport
  Enable : EnablePort
  Constant : Constant
  Constant1 : Constant  Value=0
  Switch : Switch  Criteria=u2 > Threshold  Threshold=0.5
  Alarm_Int : Outport  OutputWhenDisabled=reset  InitialOutput=0  VectorParamsAs1DForOutWhenUnconnected=off
  wires:
  "Time "/1 -> Switch/2
  Constant/1 -> Switch/1
  Constant1/1 -> Switch/3
  Switch/1 -> Alarm_Int/1

== system Aenea_model/AUTOPILOT_MODEL/AUTOPILOTA/GESTIONE AUTOPILOTI1/Intervento Manager/Alarm_Timing_0.5sec/Resettable Subsystem ==
  Reset : ResetPort  DisableCoverage=on
  CLOCK : Subsystem
  Time : Outport  VectorParamsAs1DForOutWhenUnconnected=off
  wires:
  CLOCK/1(Time) -> Time/1

== system Aenea_model/AUTOPILOT_MODEL/AUTOPILOTA/GESTIONE AUTOPILOTI1/Intervento Manager/Alarm_Timing_1sec/Enabled  ==
  "Time " : Inport
  Enable : EnablePort
  Constant : Constant
  Constant1 : Constant  Value=0
  Switch : Switch  Criteria=u2 > Threshold  Threshold=1
  Alarm_Int : Outport  OutputWhenDisabled=reset  InitialOutput=0  VectorParamsAs1DForOutWhenUnconnected=off
  wires:
  "Time "/1 -> Switch/2
  Constant/1 -> Switch/1
  Constant1/1 -> Switch/3
  Switch/1 -> Alarm_Int/1

== system Aenea_model/AUTOPILOT_MODEL/AUTOPILOTA/GESTIONE AUTOPILOTI1/Intervento Manager/Alarm_Timing_1sec/Resettable Subsystem ==
  Reset : ResetPort  DisableCoverage=on
  CLOCK : Subsystem
  Time : Outport  VectorParamsAs1DForOutWhenUnconnected=off
  wires:
  CLOCK/1(Time) -> Time/1

== system Aenea_model/AUTOPILOT_MODEL/AUTOPILOTA/GESTIONE AUTOPILOTI1/Safe Manager/Alarm_Timing/Enabled  ==
  "Time " : Inport
  Enable : EnablePort
  Constant : Constant
  Constant1 : Constant  Value=0
  Switch : Switch  Criteria=u2 > Threshold  Threshold=time_alarm_SAFE
  Alarm Safe : Outport  OutputWhenDisabled=reset  InitialOutput=0  VectorParamsAs1DForOutWhenUnconnected=off
  wires:
  "Time "/1 -> Switch/2
  Constant/1 -> Switch/1
  Constant1/1 -> Switch/3
  Switch/1 -> Alarm Safe/1

== system Aenea_model/AUTOPILOT_MODEL/AUTOPILOTA/GESTIONE AUTOPILOTI1/Safe Manager/Alarm_Timing/Resettable Subsystem ==
  Reset : ResetPort  DisableCoverage=on
  CLOCK : Subsystem
  Time : Outport  VectorParamsAs1DForOutWhenUnconnected=off
  wires:
  CLOCK/1(Time) -> Time/1

== system Aenea_model/AUTOPILOT_MODEL/AUTOPILOTA/Subsystem1/Subsystem1/LLA to Flat Earth/Subsystem1 ==
  pos_rad : Inport
  mu : Inport  Port=2
  psi_ref : Inport  Port=3
  Demux : Demux  Outputs=2
  SinCos : Trigonometry  Operator=sincos
  Subsystem : Subsystem
  Sum2 : Sum  Inputs=|++
  Sum3 : Sum  Inputs=|-+
  dEast : Product  Inputs=/*  RndMeth=Zero
  dNorth : Product  Inputs=*/  RndMeth=Zero
  x*cos : Product  RndMeth=Zero
  x*sin : Product  RndMeth=Zero
  y*cos : Product  RndMeth=Zero
  y*sin : Product  RndMeth=Zero
  Px : Outport  VectorParamsAs1DForOutWhenUnconnected=off
  Py : Outport  Port=2  VectorParamsAs1DForOutWhenUnconnected=off
  wires:
  SinCos/1 -> y*sin/2, x*sin/2
  dNorth/1 -> x*cos/1, x*sin/1
  Sum2/1 -> Px/1  "Px"
  Demux/2 -> dEast/2
  x*cos/1 -> Sum2/1
  Subsystem/2(dEast) -> dEast/1
  psi_ref/1 -> SinCos/1
  Demux/1 -> dNorth/1
  dEast/1 -> y*sin/1, y*cos/1
  Sum3/1 -> Py/1  "Py"
  y*cos/1 -> Sum3/2
  y*sin/1 -> Sum2/2
  Subsystem/1(dNorth) -> dNorth/2
  SinCos/2 -> x*cos/2, y*cos/2
  pos_rad/1 -> Demux/1
  x*sin/1 -> Sum3/1
  mu/1 -> Subsystem/1(mu)

== system Aenea_model/AUTOPILOT_MODEL/AUTOPILOTA/GESTIONE AUTOPILOTI1/Intervento Manager/Alarm_Timing_0.5sec/Resettable Subsystem/CLOCK ==
  Constant4 : Constant  Value=t_AP  SampleTime=t_AP
  Memory : Memory  InheritSampleTime=on
  Sum : Sum  Inputs=|++
  Time : Outport  VectorParamsAs1DForOutWhenUnconnected=off
  wires:
  Memory/1 -> Sum/2
  Sum/1 -> Memory/1, Time/1
  Constant4/1 -> Sum/1

== system Aenea_model/AUTOPILOT_MODEL/AUTOPILOTA/GESTIONE AUTOPILOTI1/Intervento Manager/Alarm_Timing_1sec/Resettable Subsystem/CLOCK ==
  Constant4 : Constant  Value=t_AP  SampleTime=t_AP
  Memory : Memory  InheritSampleTime=on
  Sum : Sum  Inputs=|++
  Time : Outport  VectorParamsAs1DForOutWhenUnconnected=off
  wires:
  Memory/1 -> Sum/2
  Sum/1 -> Memory/1, Time/1
  Constant4/1 -> Sum/1

== system Aenea_model/AUTOPILOT_MODEL/AUTOPILOTA/GESTIONE AUTOPILOTI1/Safe Manager/Alarm_Timing/Resettable Subsystem/CLOCK ==
  Constant4 : Constant  Value=t_AP  SampleTime=t_AP
  Memory : Memory  InheritSampleTime=on
  Sum : Sum  Inputs=|++
  Time : Outport  VectorParamsAs1DForOutWhenUnconnected=off
  wires:
  Memory/1 -> Sum/2
  Sum/1 -> Memory/1, Time/1
  Constant4/1 -> Sum/1

== system Aenea_model/AUTOPILOT_MODEL/AUTOPILOTA/Subsystem1/Subsystem1/LLA to Flat Earth/Subsystem1/Subsystem ==
  mu : Inport
  Constant : Constant  SampleTime=0.02
  Constant1 : Constant  Value=6378137  SampleTime=0.02
  Constant2 : Constant  SampleTime=0.02
  Constant3 : Constant
  Degrees to Radians : simulink_extras/Transformations/Degrees to Radians
  Product1 : Product  Inputs=*/  RndMeth=Zero
  Product2 : Product  RndMeth=Zero
  Product3 : Product  Inputs=**/  RndMeth=Zero
  Product4 : Product  RndMeth=Zero
  Subsystem : Subsystem
  Subsystem1 : Subsystem
  Sum1 : Sum  Inputs=|+-
  Trigonometric Function : Trigonometry  Operator=cos
  Trigonometric Function1 : Trigonometry  Operator=atan2
  Trigonometric Function2 : Trigonometry  Operator=atan2
  denom : aerolibtransform2/LLA to Flat Earth/Subsystem/Find Radian//Distance/denom  SystemSampleTime=-1  VariantActivationTime=update diagram  Latency=0  AutoFrameSizeCalculation=off
      settings: SourceProductBaseCode=AE
  e^1 : aerolibtransform2/Geocentric to  Geodetic Latitude/e^4  Commented=on  SystemSampleTime=-1
      settings: SourceProductBaseCode=AE
  sqrt : Sqrt  AlgorithmType=Newton-Raphson  SaturateOnIntegerOverflow=on
  dNorth : Outport  VectorParamsAs1DForOutWhenUnconnected=off
  dEast : Outport  Port=2  VectorParamsAs1DForOutWhenUnconnected=off
  wires:
  Constant2/1 -> Trigonometric Function1/1
  Constant1/1 -> Product1/1
  Product4/1 -> Trigonometric Function2/2
  Trigonometric Function/1 -> Product4/2
  Product3/1 -> Trigonometric Function1/2  "Rm"
  Subsystem/1(e) -> Subsystem1/1(e)
  Constant3/1 -> Trigonometric Function2/1
  Trigonometric Function1/1 -> dNorth/1
  Trigonometric Function2/1 -> dEast/1
  Product1/1 -> Product3/1, Product4/1  "Rn"
  denom/1 -> Product3/3, sqrt/1
  mu/1 -> Degrees to Radians/1
  Sum1/1 -> Product3/2
  Subsystem1/1(eps) -> denom/1, Product2/1, Product2/2
  Degrees to Radians/1 -> denom/2, Trigonometric Function/1
  Constant/1 -> Sum1/1
  sqrt/1 -> Product1/2
  Product2/1 -> Sum1/2

== system Aenea_model/AUTOPILOT_MODEL/AUTOPILOTA/Subsystem1/Subsystem1/LLA to Flat Earth/Subsystem1/Subsystem/Subsystem ==
  Constant : Constant  Value=1/298.257223563  SampleTime=0.02
  Sum : Sum  Inputs=-+
  f : Constant  SampleTime=0.02
  e : Outport  VectorParamsAs1DForOutWhenUnconnected=off
  wires:
  Constant/1 -> Sum/1
  f/1 -> Sum/2
  Sum/1 -> e/1

== system Aenea_model/AUTOPILOT_MODEL/AUTOPILOTA/Subsystem1/Subsystem1/LLA to Flat Earth/Subsystem1/Subsystem/Subsystem1 ==
  e : Inport
  Constant4 : Constant
  Product : Product
  Sqrt : Sqrt  SaturateOnIntegerOverflow=on
  Sum : Sum  Inputs=+-
  eps : Outport
  wires:
  Product/1 -> Sum/2
  Sqrt/1 -> eps/1
  e/1 -> Product/2, Product/1
  Constant4/1 -> Sum/1
  Sum/1 -> Sqrt/1

== stateflow chart Aenea_model/AUTOPILOT_MODEL/AUTOPILOTA/Subsystem1/DECOLLO AUTOMATICO/Chart1 ==
  state Fase_0_ATO
    du:
    Fase_ATO = 0;
    psi_ref_selector = 0;
    theta_ground_selector = 0;
    psi_ref = 0;
    phi_ref = 0;
    eq_rot = 0;
    Tas_ref = 0;
    pitch_ref = 0;
    h_ref = 0;
  state Fase_2_ATO %rullaggio
    du:
    Fase_ATO = 2;
    % devo mettere uno switch sulla manetta che tramite FASE_ATO la incrementa gradualmente fino al massimo e poi switcho sul controllore di velocita
    psi_ref_selector=0;
    psi_ref = psi_hold;
    phi_ref = 0;
    h_ref = 0;
    eq_rot = 2;
    Tas_ref = 25;
  note: la condizione V_>10 va messa soltanto in HIL, altrimenti in presenza di vento simulato l'aereo non parte
  state Fase_1_ATO
    du:
    Fase_ATO = 1;
    manetta_ref = 0.1;
    psi_ref_selector=0;
    h_ref = 0;
    psi_ref = psi_hold;
    phi_ref = 0;
    eq_rot = 2;
  state Fase_3_ATO  %rotazione
    du:
    Fase_ATO = 3;
    psi_ref_selector=0;
    theta_ground_selector = 0;
    psi_ref = psi_hold;
    phi_ref = 0;
    h_ref = 0;
    pitch_ref = 10 + theta_ground_hold;
    Tas_ref = 25;
    %devo passare al controllore di pitch, prima davo direttamente l'angolo dell'equilibratore a picchiare (ora devo fare la rotazione)
  note: quando si carica su arduino mettere manetta_ref = 0.05
      | o leggermente piu alto, in modo che l'elica giri ma non spinga
  state Fase_4_ATO  %salita
    du:
    Fase_ATO = 4;
    psi_ref_selector=0;
    psi_ref = psi_hold;
    h_ref = 35;
    RC_ref = 3;
    Tas_ref = 25;
    %devo passare al controllore di quota, prima controllavo il pitch
    %devo passare al controllore di roll canonico, prima fissavo il riferimento di roll = 0
  (default) -> Fase_0_ATO
  Fase_0_ATO -> Fase_1_ATO : [modo==3]{psi_ref_selector=1;}
  Fase_2_ATO %rullaggio -> Fase_3_ATO  %rotazione : [TAS >= 18 && V_ >= 10]{theta_ground_selector = 1;}
  Fase_1_ATO -> Fase_2_ATO %rullaggio : after(250,tick)
  Fase_3_ATO  %rotazione -> Fase_4_ATO  %salita : [h >= 2]
  Fase_4_ATO  %salita -> (junction 67)
  data: modo input; Fase_ATO output; manetta_ref output; psi_ref output; eq_rot output; phi_ref output; TAS input; pitch_ref output; h_ref output; Tas_ref output; h input; psi_hold input; RC_ref output; psi_ref_selector output; theta_ground_selector output; theta_ground_hold input; V_ input

== matlab function Aenea_model/AUTOPILOT_MODEL/AUTOPILOTA/Subsystem1/Subsystem1/APPROACH/MATLAB Function ==
  data: reset input; gamma input; x_f_out output; h_f_out output; xg0 input; k_x_out output; h_c_out output; no_solution output
function [x_f_out,h_f_out,k_x_out,h_c_out,no_solution] = fcn(reset,gamma,xg0)

 

x_f=-200;
h_f=1.5;
%x_f=-300;
%h_f=10;
k_x=0.01;
h_c=-2;
x_td=5;
h_td_dot=-0.1;
x_td_dot=18;
no_solution = 0;

% x_f=-200;
% h_f=5;
% %x_f=-300;
% %h_f=10;
% k_x=0.01;
% h_c=-1;
% x_td=50;
% h_td_dot=-0.15;
% x_td_dot=18;
% no_solution = 0;

% F = [f(x_f,h_f,gamma,xg0); g(h_c,h_f,k_x,gamma); r(h_c,h_f,k_x,x_f,x_td); s(h_c,h_f,k_x,x_f,x_td,h_td_dot,x_td_dot)];
% 
% J = [ df1() df2(gamma) df3() df4();
%       dg1(k_x) dg2() dg3(h_f,h_c) dg4(k_x);
%       dr1(k_x,x_td,x_f) dr2(k_x,x_td,x_f) dr3(k_x,x_td,x_f,h_f,h_c) dr4();
%       ds1(k_x,x_td,x_f,x_td_dot) ds2(k_x,x_td,x_f,x_td_dot,h_f,h_c) ds3(k_x,x_td,x_f,x_td_dot,h_f,h_c) ds4(k_x,x_td,x_f,x_td_dot)]

persistent x x_new cycle_count eps

if (isempty(x) ||  reset == 0)
x = [h_f; x_f; k_x; h_c];
end

if (isempty(x_new) || reset == 0)
x_new = zeros(4,1);
end

if (isempty(eps) || reset == 0)
eps = ones(1,4);
end
   
if (isempty(cycle_count) || reset == 0)
cycle_count = 0;
end




while ~ (eps(1) < 0.1 && eps(2) < 0.1 && eps(3) < 0.1 && eps(4) < 0.1 )

F = [f(x(2),x(1),gamma,xg0); g(x(4),x(1),x(3),gamma); r(x(4),x(1),x(3),x(2),x_td); s(x(4),x(1),x(3),x(2),x_td,h_td_dot,x_td_dot)];

J = [ df1() df2(gamma) df3() df4();
      dg1(x(3)) dg2() dg3(x(1),x(4)) dg4(x(3));
      dr1(x(3),x_td,x(2)) dr2(x(3),x_td,x(2),x(1),x(4)) dr3(x(3),x_td,x(2),x(1),x(4)) dr4();
      ds1(x(3),x_td,x(2),x_td_dot) ds2(x(3),x_td,x(2),x_td_dot,x(1),x(4)) ds3(x(3),x_td,x(2),x_td_dot,x(1),x(4)) ds4(x(3),x_td,x(2),x_td_dot)] ; 
  
  
x_new = x - J^(-1)*F;

eps(1) = abs(x_new(1)-x(1));
eps(2) = abs(x_new(2)-x(2));
eps(3) = abs(x_new(3)-x(3));
eps(4) = abs(x_new(4)-x(4));


x = x_new;

cycle_count = cycle_count + 1;

if cycle_count > 10
   no_solution = 1; 
   break; 
end

end

if (eps(1) < 0.1 && eps(2) < 0.1 && eps(3) < 0.1 && eps(4) < 0.1 )
   
h_f_out = x(1);
x_f_out = x(2);
k_x_out = x(3);
h_c_out = x(4);

else
    
h_f_out = 0;
x_f_out = 0;
k_x_out = 0;
h_c_out = 0;    
end

function y = f(x_f,h_f,gamma,xg0)                 %inizio equazioni sistema non lineare
y = h_f+(x_f-xg0)*tan(gamma);
end

function y = g(h_c,h_f,k_x,gamma)
y = (h_f-h_c)*k_x-tan(gamma);
end

function y = r(h_c,h_f,k_x,x_f,x_td)
y = h_c + (h_f-h_c)*exp(-k_x*(x_td-x_f));
end

function y = s(h_c,h_f,k_x,x_f,x_td,h_td_dot,x_td_dot)
y = h_td_dot + (h_f-h_c)*k_x*x_td_dot*exp(-k_x*(x_td-x_f));        
end                                                                   % fine equazioni sistema non lineare

function y = df1()                                                    %inizio derivate
y = 1;
end

function y = df2(gamma)
y = tan(gamma);
end

function y = df3()
y = 0;
end

function y = df4()
y = 0;
end

function y = dg1(k_x)
y = k_x;
end

function y = dg2()
y = 0;
end

function y = dg3(h_f,h_c)
y = h_f-h_c;
end

function y = dg4(k_x)
y = -k_x;
end

function y = dr1(k_x,x_td,x_f)
y = exp(-k_x*(x_td-x_f));
end

function y = dr2(k_x,x_td,x_f,h_f,h_c)
y = (h_f-h_c)*k_x*exp(-k_x*(x_td-x_f));
end

function y = dr3(k_x,x_td,x_f,h_f,h_c)
y = (h_f-h_c)*(x_f-x_td)*exp(-k_x*(x_td-x_f));
end

function y = dr4()
y = 1;
end

function y = ds1(k_x,x_td,x_f,x_td_dot)
y = k_x*x_td_dot*exp(-k_x*(x_td-x_f));
end

function y = ds2(k_x,x_td,x_f,x_td_dot,h_f,h_c)
y = (h_f-h_c)*k_x^2*x_td_dot*exp(-k_x*(x_td-x_f));
end

function y = ds3(k_x,x_td,x_f,x_td_dot,h_f,h_c)
y = (h_f-h_c)*x_td_dot*exp(-k_x*(x_td-x_f))+(h_f-h_c)*k_x*x_td_dot*(x_f-x_td)*exp(-k_x*(x_td-x_f));
end

function y = ds4(k_x,x_td,x_f,x_td_dot)
y = -k_x*x_td_dot*exp(-k_x*(x_td-x_f));
end



end

== matlab function Aenea_model/AUTOPILOT_MODEL/Misure Sensori/BMP_280/MATLAB Function ==
  data: rate_l_up output; Cal_alt input; P input; P_int input; P_refer output; P_cal input; rate_l_dw output
function [rate_l_up, P_refer, rate_l_dw]  = fcn( Cal_alt, P,P_int,P_cal)
%#codegen

persistent P_ref rl_up rl_dw

if isempty(P_ref)
    
    P_ref = 102600; %101440
    
end

if isempty(rl_up)
    
    rl_up = 300;
    
end

if isempty(rl_dw)
    
    rl_dw = -300;
    
end

if Cal_alt == 1
    
    P_ref = P;
 
end

if P_int == 1
   
   P_ref = P_cal; 
   rl_up = 20;
   rl_dw = -20;
    
end
    


P_refer = P_ref;

rate_l_up = rl_up;
rate_l_dw = rl_dw;

== matlab function Aenea_model/AUTOPILOT_MODEL/Misure Sensori/MTi/MATLAB Function1 ==
  data: messaggio input; Mex_out output; Mex_prec input; Control output
function [Mex_out,Control]  = checksum_control(messaggio,Mex_prec)

Control = uint8(0);

mti_string = uint8(messaggio(2:41));

checksum = sum(mti_string) ; 

hex_checksum = dec2hex(checksum);

if ((hex_checksum(3) == '0') && (hex_checksum(4) == '0'))
    Mex_out = uint8(messaggio);

else
   Control = uint8(1); 
   Mex_out = Mex_prec;   
end



end
